simulink model "robot_model2b"  (R2020b)
settings: Solver=ode4  StartTime=0.0  StopTime=50  FixedStep=T_s  RelTol=1e-3  EnableMultiTasking=on
InitFcn:
  | init_exp_icr
values from neighbouring files (symbols this model uses):
  g = 9.81    [init_exp_icr.m]
  K = [constx;consty;consttheta]    [init_exp_icr.m]
  l1 = 1    [init_exp_icr.m]
  lc1 = l1/2    (= 0.5)    [init_exp_icr.m]
  lc2 = l2/2    (= 0.5)    [init_exp_icr.m]
  m1 = 1    [init_exp_icr.m]
  m2 = 1    [init_exp_icr.m]
undefined symbols (not defined in the file or in its folder): I1zz, I2zz
settings Model: Creator=Lars  LastModifiedBy=jsol
settings SolverCC: AutoInsertRateTranBlk=on
settings DataIOCC: LimitDataPoints=on  SaveFormat=Array  ReturnWorkspaceOutputs=off
settings OptimizationCC: LifeSpan=inf
settings DebuggingCC: UnderspecifiedInitializationDetection=Classic  MergeDetectMultiDrivingBlocksExec=none  SolverPrmCheckMsg=warning  AllowSymbolicDim=off  SFUnexpectedBacktrackingDiag=warning  SFNoUnconditionalDefaultTransitionDiag=warning  SFExecutionAtInitializationDiag=none  ArithmeticOperatorsInVariantConditions=warning
settings HardwareCC: ProdBitPerPointer=32  ProdBitPerSizeT=32  ProdBitPerPtrDiffT=32  ProdLargestAtomicFloat=None  ProdIntDivRoundTo=Undefined  ProdEndianess=Unspecified  ProdWordSize=32  ProdHWDeviceType=32-bit Generic
settings ModelReferenceCC: PropagateSignalLabelsOutOfModel=off
settings SFSimCC: SimUseLocalCustomCode=off  CustomCodeUndefinedFunction=UseInterfaceOnly
settings RTWCC: RTWUseLocalCustomCode=off
settings CodeAppCC: StateflowObjectComments=on
settings GRTTargetCC: TargetLangStandard=C89/C90 (ANSI)
settings ConfigComp: CovMetricSettings=dw  CovSaveCumulativeToWorkspaceVar=on  CovSaveSingleToWorkspaceVar=on  CovExternalEMLEnable=off

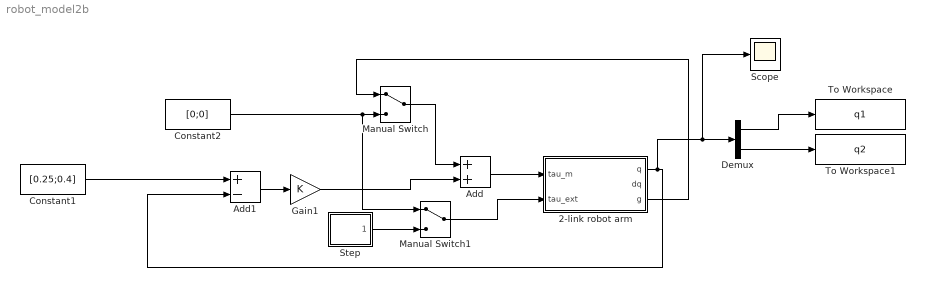
== system robot_model2b ==
  2-link robot arm : Subsystem
  Add : Sum
  Add1 : Sum  Inputs=+-
  Constant1 : Constant  Value=[0.25;0.4]
  Constant2 : Constant  Value=[0;0]
  Demux : Demux  Outputs=2
  Gain1 : Gain  Gain=K
  Manual Switch : ManualSwitch
  Manual Switch1 : ManualSwitch
  Scope : Scope
  Step : Subsystem
  To Workspace : ToWorkspace  VariableName=q1  SaveFormat=Timeseries  SampleTime=-1
  To Workspace1 : ToWorkspace  VariableName=q2  SaveFormat=Timeseries  SampleTime=-1
  wires:
  2-link robot arm/1("q ") -> Scope/1, Demux/1, Add1/2
  Demux/1 -> To Workspace/1
  Demux/2 -> To Workspace1/1
  Add/1 -> 2-link robot arm/1(tau_m)
  2-link robot arm/3(g) -> Manual Switch/1
  Manual Switch/1 -> Add/1
  Constant2/1 -> Manual Switch1/1, Manual Switch/2
  Constant1/1 -> Add1/1
  Add1/1 -> Gain1/1
  Gain1/1 -> Add/2
  Step/1(tau_ext) -> Manual Switch1/2
  Manual Switch1/1 -> 2-link robot arm/2(tau_ext)

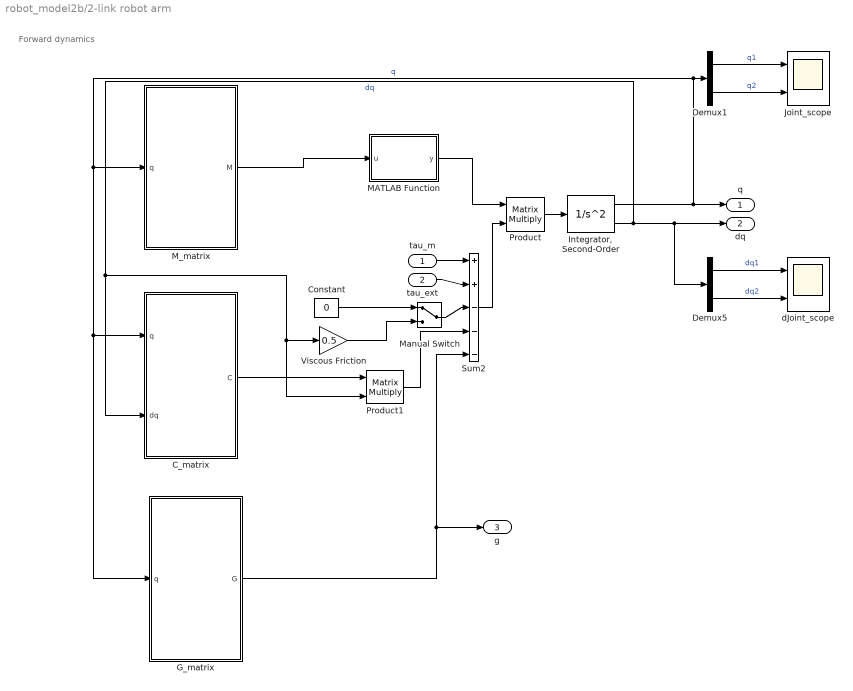
== system robot_model2b/2-link robot arm ==
  note: Forward dynamics
  tau_m : Inport
  tau_ext : Inport  Port=2
  C_matrix : MATLAB Function  TreatAsAtomicUnit=on
  Constant : Constant  Value=0
  Demux1 : Demux  Outputs=2
  Demux5 : Demux  Outputs=2
  G_matrix : MATLAB Function  TreatAsAtomicUnit=on
  "Integrator, Second-Order" : SecondOrderIntegrator  ICX=[0,0]  ICDXDT=[0 0]
  Joint_scope : Scope  NumInputPorts=2
  MATLAB Function : MATLAB Function  TreatAsAtomicUnit=on
  M_matrix : MATLAB Function  TreatAsAtomicUnit=on
  Manual Switch : ManualSwitch
  Product : Product  Multiplication=Matrix(*)
  Product1 : Product  Multiplication=Matrix(*)
  Sum2 : Sum  Inputs=++|---
  Viscous Friction : Gain  Gain=0.5
  dJoint_scope : Scope  NumInputPorts=2
  "q " : Outport
  "dq " : Outport  Port=2
  g : Outport  Port=3
  wires:
  Demux1/1 -> Joint_scope/1  "q1"
  Demux1/2 -> Joint_scope/2  "q2"
  "Integrator, Second-Order"/2 -> Demux5/1, "dq "/1, Product1/2, Viscous Friction/1, C_matrix/2(dq)  "dq"
  Demux5/1 -> dJoint_scope/1  "dq1"
  C_matrix/1(C) -> Product1/1
  "Integrator, Second-Order"/1 -> "q "/1, Demux1/1, G_matrix/1(q), C_matrix/1(q), M_matrix/1(q)  "q"
  Demux5/2 -> dJoint_scope/2  "dq2"
  Sum2/1 -> Product/2
  Constant/1 -> Manual Switch/1
  Viscous Friction/1 -> Manual Switch/2
  M_matrix/1(M) -> MATLAB Function/1(u)
  Product/1 -> "Integrator, Second-Order"/1
  G_matrix/1(G) -> Sum2/5, g/1
  Product1/1 -> Sum2/4
  Manual Switch/1 -> Sum2/3
  tau_m/1 -> Sum2/1
  tau_ext/1 -> Sum2/2
  MATLAB Function/1(y) -> Product/1

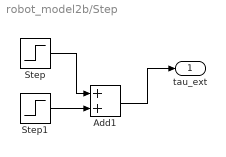
== system robot_model2b/Step ==
  Add1 : Sum
  Step : Step  Time=5  Before=[0;0]  After=[0.5;3]  SampleTime=0
  Step1 : Step  Time=5.2  Before=[0;0]  After=[-0.5;-3]  SampleTime=0
  tau_ext : Outport
  wires:
  Step1/1 -> Add1/2
  Step/1 -> Add1/1
  Add1/1 -> tau_ext/1

== matlab function robot_model2b/2-link robot arm/C_matrix ==
  data: q input; C output; dq input; l1 parameter; lc2 parameter; m2 parameter
function C = C_matrix(q,dq, l1, lc2, m2)
%#codegen

%    This function was generated by the Symbolic Math Toolbox version 8.3.
%    05-Nov-2019 15:18:30
q1 = q(1);
q2 = q(2);
dq1 = dq(1);
dq2 = dq(2);
t2 = sin(q2);
C = reshape([-dq2.*l1.*lc2.*m2.*t2,dq1.*l1.*lc2.*m2.*t2,-l1.*lc2.*m2.*t2.*(dq1+dq2),0.0],[2,2]);

== matlab function robot_model2b/2-link robot arm/M_matrix ==
  data: M output; q input; I1zz parameter; I2zz parameter; l1 parameter; lc1 parameter; lc2 parameter; m1 parameter; m2 parameter
function M = M_matrix(q, I1zz, I2zz, l1, lc1, lc2, m1, m2)
%#codegen

%    This function was generated by the Symbolic Math Toolbox version 8.3.
%    05-Nov-2019 15:18:29
q1 = q(1);
q2 = q(2);
t2 = cos(q2);
t3 = lc2.^2;
t4 = m2.*t3;
t5 = l1.*lc2.*m2.*t2;
t6 = I2zz+t4+t5;
M = reshape([I1zz+t5+t6+l1.^2.*m2+lc1.^2.*m1,t6,t6,I2zz+t4],[2,2]);

== matlab function robot_model2b/2-link robot arm/MATLAB Function ==
  data: u input; y output
function y = inverse_matrix(u)
    if det(u) ~= 0
        y = inv(u);
    else
        y = zeros(size(u)); % or handle singular case differently
    end
end

== matlab function robot_model2b/2-link robot arm/G_matrix ==
  data: G output; q input; g parameter; l1 parameter; lc1 parameter; lc2 parameter; m1 parameter; m2 parameter
function G = G_matrix(q, g, l1, lc1, lc2, m1, m2)
%#codegen

%    This function was generated by the Symbolic Math Toolbox version 8.3.
%    05-Nov-2019 15:18:30
q1 = q(1);
q2 = q(2);
t2 = cos(q1);
t3 = q1+q2;
t4 = cos(t3);
G = [g.*m2.*(l1.*t2+lc2.*t4)+g.*lc1.*m1.*t2;g.*lc2.*m2.*t4];
